simulink model "PrimeirOrdem"  (R2020a)
settings: Solver=VariableStepAuto  StartTime=0.0  StopTime=10  RelTol=1e-3
undefined symbols (not defined in the file): T
libraries: simulink x1
settings Model: Creator=a1  LastModifiedBy=a1

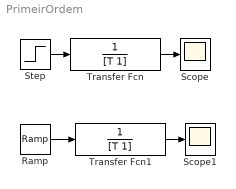
== system PrimeirOrdem ==
  Ramp : simulink/Sources/Ramp  slope=1  start=0  InitialOutput=0
  Scope : Scope
  Scope1 : Scope
  Step : Step  SampleTime=0
  Transfer Fcn : TransferFcn  Denominator=[T 1]
  Transfer Fcn1 : TransferFcn  Denominator=[T 1]
  wires:
  Step/1 -> Transfer Fcn/1
  Transfer Fcn/1 -> Scope/1
  Ramp/1 -> Transfer Fcn1/1
  Transfer Fcn1/1 -> Scope1/1
